simulink model "BLDC_Motor_System_Diagram"  (R2020a)
settings: Solver=VariableStepAuto  StartTime=0.0  StopTime=10.0  RelTol=1e-3
settings Model: Creator=Sony  LastModifiedBy=Sony

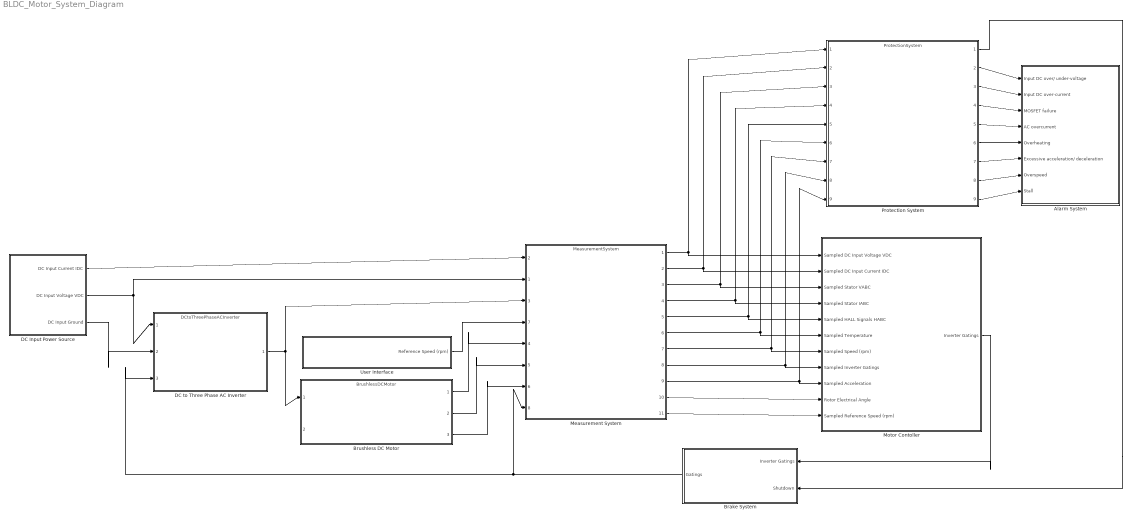
== system BLDC_Motor_System_Diagram ==
  Alarm System : Subsystem
      settings: PortSchema="{\"entries\":[{\"content\":{\"headerSize\":26,\"margin\":15,\"minimumSpacing\":25,\"sides\":[{\"content\":{\"connectorIds\":[\"In1\",\"In2\",\"In3\",\"In4\",\"In5\",\"In6\",\"In7\",\"In8\"]},\"type\":\"ConnectorPlacement.EquallySpacedRectSide\",\"uuid\":\"ace81693-b25f-4784-848a-70d4510dde11\"},{\"content\":{\"connectorIds\":[],\"side\":\"RIGHT\"},\"type\":\"ConnectorPlacement.EquallySpacedRectSide\",\"uuid\":\"ee57309e-8484-4f62-a9df-3d3bfb9210c2\"},{\"content\":{\"connectorIds\":[],\"side\":\"TOP\"},\"type\":\"ConnectorPlacement.EquallySpacedRectSide\",\"uuid\":\"4da7af74-213e-40d9-8573-ef4a383eae7e\"}]},\"type\":\"ConnectorPlacement.EquallySpacedConnector\",\"uuid\":\"ce645311-a995-4bdd-afab-02a7660553a7\"}],\"packageUris\":[\"http://schema.mathworks.com/mf0/Connector/19700101\"],\"version\":\"1.0\"}"
  Brake System : Subsystem
      settings: PortSchema="{\"entries\":[{\"content\":{\"headerSize\":26,\"margin\":15,\"minimumSpacing\":25,\"sides\":[{\"content\":{\"connectorIds\":[\"Out1\"]},\"type\":\"ConnectorPlacement.EquallySpacedRectSide\",\"uuid\":\"ace81693-b25f-4784-848a-70d4510dde11\"},{\"content\":{\"connectorIds\":[\"In1\",\"In2\"],\"side\":\"RIGHT\"},\"type\":\"ConnectorPlacement.EquallySpacedRectSide\",\"uuid\":\"ee57309e-8484-4f62-a9df-3d3bfb9210c2\"},{\"content\":{\"connectorIds\":[],\"side\":\"TOP\"},\"type\":\"ConnectorPlacement.EquallySpacedRectSide\",\"uuid\":\"4da7af74-213e-40d9-8573-ef4a383eae7e\"}]},\"type\":\"ConnectorPlacement.EquallySpacedConnector\",\"uuid\":\"ce645311-a995-4bdd-afab-02a7660553a7\"}],\"packageUris\":[\"http://schema.mathworks.com/mf0/Connector/19700101\"],\"version\":\"1.0\"}"
  Brushless DC Motor : ModelReference  ModelNameDialog=BrushlessDCMotor  SimulationMode=Normal  ModelReferenceVersion=1.5
      settings: PortSchema="{\"entries\":[{\"content\":{\"headerSize\":38,\"margin\":15,\"minimumSpacing\":25,\"sides\":[{\"content\":{\"connectorIds\":[\"In1\",\"In2\"]},\"type\":\"ConnectorPlacement.EquallySpacedRectSide\",\"uuid\":\"ace81693-b25f-4784-848a-70d4510dde11\"},{\"content\":{\"connectorIds\":[\"Out1\",\"Out2\",\"Out3\"],\"side\":\"RIGHT\"},\"type\":\"ConnectorPlacement.EquallySpacedRectSide\",\"uuid\":\"ee57309e-8484-4f62-a9df-3d3bfb9210c2\"},{\"content\":{\"connectorIds\":[],\"side\":\"TOP\"},\"type\":\"ConnectorPlacement.EquallySpacedRectSide\",\"uuid\":\"4da7af74-213e-40d9-8573-ef4a383eae7e\"}]},\"type\":\"ConnectorPlacement.EquallySpacedConnector\",\"uuid\":\"ce645311-a995-4bdd-afab-02a7660553a7\"}],\"packageUris\":[\"http://schema.mathworks.com/mf0/Connector/19700101\"],\"version\":\"1.0\"}"
  DC Input Power Source : Subsystem
      settings: PortSchema="{\"entries\":[{\"content\":{\"headerSize\":26,\"margin\":15,\"minimumSpacing\":25,\"sides\":[{\"content\":{\"connectorIds\":[]},\"type\":\"ConnectorPlacement.EquallySpacedRectSide\",\"uuid\":\"ace81693-b25f-4784-848a-70d4510dde11\"},{\"content\":{\"connectorIds\":[\"Out1\",\"Out2\",\"Out3\"],\"side\":\"RIGHT\"},\"type\":\"ConnectorPlacement.EquallySpacedRectSide\",\"uuid\":\"ee57309e-8484-4f62-a9df-3d3bfb9210c2\"},{\"content\":{\"connectorIds\":[],\"side\":\"TOP\"},\"type\":\"ConnectorPlacement.EquallySpacedRectSide\",\"uuid\":\"4da7af74-213e-40d9-8573-ef4a383eae7e\"}]},\"type\":\"ConnectorPlacement.EquallySpacedConnector\",\"uuid\":\"ce645311-a995-4bdd-afab-02a7660553a7\"}],\"packageUris\":[\"http://schema.mathworks.com/mf0/Connector/19700101\"],\"version\":\"1.0\"}"
  DC to Three Phase AC Inverter : ModelReference  ModelNameDialog=DCtoThreePhaseACInverter  SimulationMode=Normal  ModelReferenceVersion=1.5
      settings: PortSchema="{\"entries\":[{\"content\":{\"headerSize\":38,\"margin\":15,\"minimumSpacing\":25,\"sides\":[{\"content\":{\"connectorIds\":[\"In1\",\"In2\",\"In3\"]},\"type\":\"ConnectorPlacement.EquallySpacedRectSide\",\"uuid\":\"ace81693-b25f-4784-848a-70d4510dde11\"},{\"content\":{\"connectorIds\":[\"Out1\"],\"side\":\"RIGHT\"},\"type\":\"ConnectorPlacement.EquallySpacedRectSide\",\"uuid\":\"ee57309e-8484-4f62-a9df-3d3bfb9210c2\"},{\"content\":{\"connectorIds\":[],\"side\":\"TOP\"},\"type\":\"ConnectorPlacement.EquallySpacedRectSide\",\"uuid\":\"4da7af74-213e-40d9-8573-ef4a383eae7e\"}]},\"type\":\"ConnectorPlacement.EquallySpacedConnector\",\"uuid\":\"ce645311-a995-4bdd-afab-02a7660553a7\"}],\"packageUris\":[\"http://schema.mathworks.com/mf0/Connector/19700101\"],\"version\":\"1.0\"}"
  Measurement System : ModelReference  ModelNameDialog=MeasurementSystem  SimulationMode=Normal  ModelReferenceVersion=1.6
      settings: PortSchema="{\"entries\":[{\"content\":{\"headerSize\":38,\"margin\":15,\"minimumSpacing\":25,\"sides\":[{\"content\":{\"connectorIds\":[\"In2\",\"In1\",\"In3\",\"In7\",\"In4\",\"In5\",\"In6\",\"In8\"]},\"type\":\"ConnectorPlacement.EquallySpacedRectSide\",\"uuid\":\"ace81693-b25f-4784-848a-70d4510dde11\"},{\"content\":{\"connectorIds\":[\"Out1\",\"Out2\",\"Out3\",\"Out4\",\"Out5\",\"Out6\",\"Out7\",\"Out8\",\"Out9\",\"Out10\",\"Out11\"],\"side\":\"RIGHT\"},\"type\":\"ConnectorPlacement.EquallySpacedRectSide\",\"uuid\":\"ee57309e-8484-4f62-a9df-3d3bfb9210c2\"},{\"content\":{\"connectorIds\":[],\"side\":\"TOP\"},\"type\":\"ConnectorPlacement.EquallySpacedRectSide\",\"uuid\":\"4da7af74-213e-40d9-8573-ef4a383eae7e\"},{\"content\":{\"connectorIds\":[],\"side\":\"BOTTOM\"},\"type\":\"ConnectorPlacement.EquallySpacedRectSide\",\"uuid\":\"d9a97e9f-44d9-4606-a897-cff504073fb6\"}]},\"type\":\"ConnectorPlacement.EquallySpacedConnector\",\"uuid\":\"ce645311-a995-4bdd-afab-02a7660553a7\"}],\"packageUris\":[\"http://schema.mathworks.com/mf0/Connector/19700101\"],\"version\":\"1.0\"}"
  Motor Contoller : Subsystem
      settings: PortSchema="{\"entries\":[{\"content\":{\"headerSize\":26,\"margin\":15,\"minimumSpacing\":25,\"sides\":[{\"content\":{\"connectorIds\":[\"In1\",\"In2\",\"In3\",\"In4\",\"In5\",\"In6\",\"In7\",\"In8\",\"In9\",\"In10\",\"In11\"]},\"type\":\"ConnectorPlacement.EquallySpacedRectSide\",\"uuid\":\"ace81693-b25f-4784-848a-70d4510dde11\"},{\"content\":{\"connectorIds\":[\"Out1\"],\"side\":\"RIGHT\"},\"type\":\"ConnectorPlacement.EquallySpacedRectSide\",\"uuid\":\"ee57309e-8484-4f62-a9df-3d3bfb9210c2\"},{\"content\":{\"connectorIds\":[],\"side\":\"TOP\"},\"type\":\"ConnectorPlacement.EquallySpacedRectSide\",\"uuid\":\"4da7af74-213e-40d9-8573-ef4a383eae7e\"}]},\"type\":\"ConnectorPlacement.EquallySpacedConnector\",\"uuid\":\"ce645311-a995-4bdd-afab-02a7660553a7\"}],\"packageUris\":[\"http://schema.mathworks.com/mf0/Connector/19700101\"],\"version\":\"1.0\"}"
  Protection System : ModelReference  ModelNameDialog=ProtectionSystem  SimulationMode=Normal  ModelReferenceVersion=1.4
      settings: PortSchema="{\"entries\":[{\"content\":{\"headerSize\":38,\"margin\":15,\"minimumSpacing\":25,\"sides\":[{\"content\":{\"connectorIds\":[\"In1\",\"In2\",\"In3\",\"In4\",\"In5\",\"In6\",\"In7\",\"In8\",\"In9\"]},\"type\":\"ConnectorPlacement.EquallySpacedRectSide\",\"uuid\":\"ace81693-b25f-4784-848a-70d4510dde11\"},{\"content\":{\"connectorIds\":[\"Out1\",\"Out2\",\"Out3\",\"Out4\",\"Out5\",\"Out6\",\"Out7\",\"Out8\",\"Out9\"],\"side\":\"RIGHT\"},\"type\":\"ConnectorPlacement.EquallySpacedRectSide\",\"uuid\":\"ee57309e-8484-4f62-a9df-3d3bfb9210c2\"},{\"content\":{\"connectorIds\":[],\"side\":\"TOP\"},\"type\":\"ConnectorPlacement.EquallySpacedRectSide\",\"uuid\":\"4da7af74-213e-40d9-8573-ef4a383eae7e\"}]},\"type\":\"ConnectorPlacement.EquallySpacedConnector\",\"uuid\":\"ce645311-a995-4bdd-afab-02a7660553a7\"}],\"packageUris\":[\"http://schema.mathworks.com/mf0/Connector/19700101\"],\"version\":\"1.0\"}"
  User Interface : Subsystem
      settings: PortSchema="{\"entries\":[{\"content\":{\"headerSize\":26,\"margin\":15,\"minimumSpacing\":25,\"sides\":[{\"content\":{\"connectorIds\":[]},\"type\":\"ConnectorPlacement.EquallySpacedRectSide\",\"uuid\":\"ace81693-b25f-4784-848a-70d4510dde11\"},{\"content\":{\"connectorIds\":[\"Out1\"],\"side\":\"RIGHT\"},\"type\":\"ConnectorPlacement.EquallySpacedRectSide\",\"uuid\":\"ee57309e-8484-4f62-a9df-3d3bfb9210c2\"},{\"content\":{\"connectorIds\":[],\"side\":\"TOP\"},\"type\":\"ConnectorPlacement.EquallySpacedRectSide\",\"uuid\":\"4da7af74-213e-40d9-8573-ef4a383eae7e\"}]},\"type\":\"ConnectorPlacement.EquallySpacedConnector\",\"uuid\":\"ce645311-a995-4bdd-afab-02a7660553a7\"}],\"packageUris\":[\"http://schema.mathworks.com/mf0/Connector/19700101\"],\"version\":\"1.0\"}"
  wires:
  DC Input Power Source/2(DC Input Voltage VDC) -> DC to Three Phase AC Inverter/1, Measurement System/1
  Motor Contoller/1(Inverter Gatings) -> Brake System/1(Inverter Gatings)
  Brake System/1(Gatings) -> DC to Three Phase AC Inverter/3, Measurement System/8
  DC Input Power Source/3(DC Input Ground) -> DC to Three Phase AC Inverter/2
  DC to Three Phase AC Inverter/1 -> Measurement System/3, Brushless DC Motor/1
  Brushless DC Motor/1 -> Measurement System/4
  Brushless DC Motor/2 -> Measurement System/5
  User Interface/1(Reference Speed (rpm)) -> Measurement System/7
  Brushless DC Motor/3 -> Measurement System/6
  Measurement System/9 -> Motor Contoller/9(Sampled Acceleration), Protection System/9
  Measurement System/2 -> Motor Contoller/2(Sampled DC Input Current IDC), Protection System/2
  Measurement System/1 -> Motor Contoller/1(Sampled DC Input Voltage VDC), Protection System/1
  Measurement System/5 -> Motor Contoller/5(Sampled HALL Signals HABC), Protection System/5
  Measurement System/8 -> Motor Contoller/8(Sampled Inverter Gatings), Protection System/8
  Measurement System/11 -> Motor Contoller/11(Sampled Reference Speed (rpm))
  Measurement System/10 -> Motor Contoller/10(Rotor Electrical Angle)
  Measurement System/7 -> Motor Contoller/7(Sampled Speed (rpm)), Protection System/7
  Measurement System/4 -> Motor Contoller/4(Sampled Stator IABC), Protection System/4
  Measurement System/3 -> Motor Contoller/3(Sampled Stator VABC), Protection System/3
  Measurement System/6 -> Motor Contoller/6(Sampled Temperature), Protection System/6
  DC Input Power Source/1(DC Input Current IDC) -> Measurement System/2
  Protection System/5 -> Alarm System/4(AC overcurrent)
  Protection System/7 -> Alarm System/6(Excessive acceleration/ deceleration)
  Protection System/3 -> Alarm System/2(Input DC over-current)
  Protection System/2 -> Alarm System/1("Input DC over/ under-voltage ")
  Protection System/4 -> Alarm System/3(MOSFET failure)
  Protection System/6 -> Alarm System/5(Overheating)
  Protection System/8 -> Alarm System/7(Overspeed)
  Protection System/1 -> Brake System/2(Shutdown)
  Protection System/9 -> Alarm System/8(Stall)

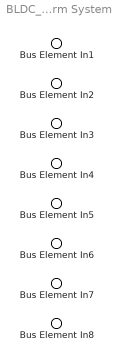
== system BLDC_Motor_System_Diagram/Alarm System ==
  Bus Element In1 : Inport  PortName=Input DC over/ under-voltage
  Bus Element In2 : Inport  Port=2  PortName=Input DC over-current
  Bus Element In3 : Inport  Port=3  PortName=MOSFET failure
  Bus Element In4 : Inport  Port=4  PortName=AC overcurrent
  Bus Element In5 : Inport  Port=5  PortName=Overheating
  Bus Element In6 : Inport  Port=6  PortName=Excessive acceleration/ deceleration
  Bus Element In7 : Inport  Port=7  PortName=Overspeed
  Bus Element In8 : Inport  Port=8  PortName=Stall

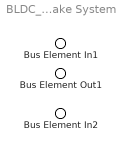
== system BLDC_Motor_System_Diagram/Brake System ==
  Bus Element In1 : Inport  PortName=Inverter Gatings
  Bus Element In2 : Inport  Port=2  PortName=Shutdown
  Bus Element Out1 : Outport  PortName=Gatings

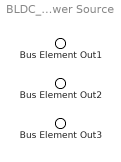
== system BLDC_Motor_System_Diagram/DC Input Power Source ==
  Bus Element Out1 : Outport  PortName=DC Input Current IDC
  Bus Element Out2 : Outport  Port=2  PortName=DC Input Voltage VDC
  Bus Element Out3 : Outport  Port=3  PortName=DC Input Ground

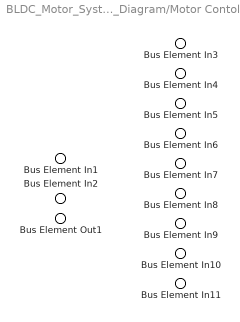
== system BLDC_Motor_System_Diagram/Motor Contoller ==
  Bus Element In1 : Inport  PortName=Sampled DC Input Voltage VDC
  Bus Element In11 : Inport  Port=2  PortName=Sampled DC Input Current IDC
  Bus Element In10 : Inport  Port=3  PortName=Sampled Stator VABC
  Bus Element In9 : Inport  Port=4  PortName=Sampled Stator IABC
  Bus Element In8 : Inport  Port=5  PortName=Sampled HALL Signals HABC
  Bus Element In7 : Inport  Port=6  PortName=Sampled Temperature
  Bus Element In6 : Inport  Port=7  PortName=Sampled Speed (rpm)
  Bus Element In5 : Inport  Port=8  PortName=Sampled Inverter Gatings
  Bus Element In4 : Inport  Port=9  PortName=Sampled Acceleration
  Bus Element In3 : Inport  Port=10  PortName=Rotor Electrical Angle
  Bus Element In2 : Inport  Port=11  PortName=Sampled Reference Speed (rpm)
  Bus Element Out1 : Outport  PortName=Inverter Gatings

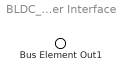
== system BLDC_Motor_System_Diagram/User Interface ==
  Bus Element Out1 : Outport  PortName=Reference Speed (rpm)
